simulink model "q1_c"  (R2023a)
settings: Solver=ode4  StartTime=0.0  StopTime=tstop  FixedStep=tstop/1000  RelTol=1e-3
libraries: cstblocks x2
settings Model: Creator=mohad  LastModifiedBy=mohad
settings DataIOCC: ReturnWorkspaceOutputs=off

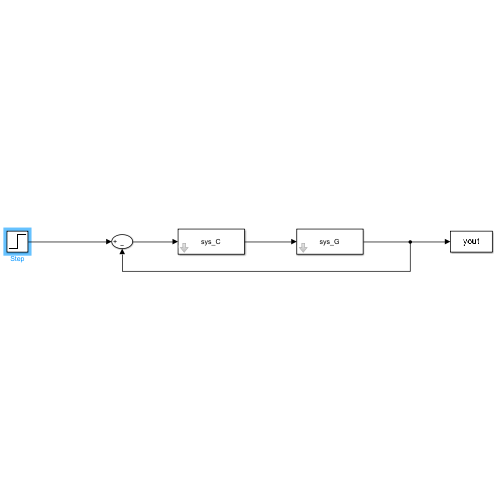
[thumbnail: Simulink's stored preview of the top-level diagram]
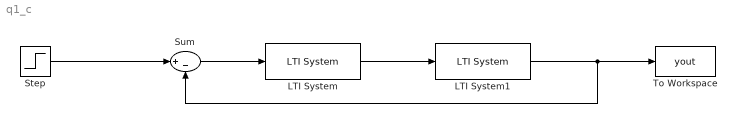
== system q1_c ==
  LTI System : cstblocks/LTI System  sys=sys_C  IC=[]
  LTI System1 : cstblocks/LTI System  sys=sys_G  IC=[]
  Step : Step  Time=0  SampleTime=0
  Sum : Sum  Inputs=|+-
  To Workspace : ToWorkspace  VariableName=yout  SampleTime=-1
  wires:
  Sum/1 -> LTI System/1
  LTI System/1 -> LTI System1/1
  LTI System1/1 -> Sum/2, To Workspace/1
  Step/1 -> Sum/1
